simulink model "ANSFT_Euler"  (R2023a)
settings: Solver=ode1  StartTime=0.0  StopTime=60  FixedStep=0.01  RelTol=1e-3
undefined symbols (not defined in the file or in its folder): HDBK, Light, MIL, sigbuilder_block
libraries: simulink x4, matrix_library x3, aerolibutil x3, robotcorelib x2, aerolibanim x1, simulink_extras x1, sharedtransform x1, aerolibwind2 x1, sim3dlib x1, uavsim3dlib x1
(part 1 of 2)
settings Model: Creator=goliv  LastModifiedBy=Adan Daniel
settings OptimizationCC: ReuseModelBlockBuffer=off

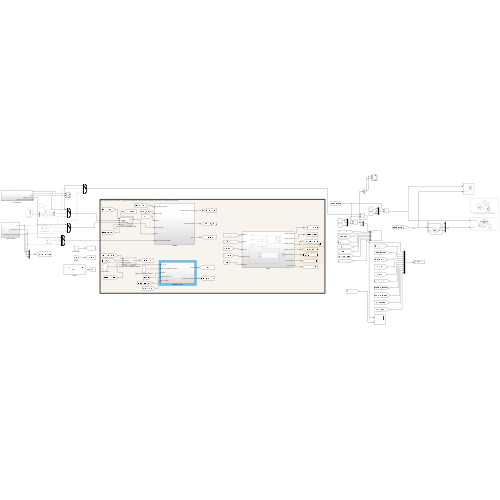
[thumbnail: Simulink's stored preview of the top-level diagram]
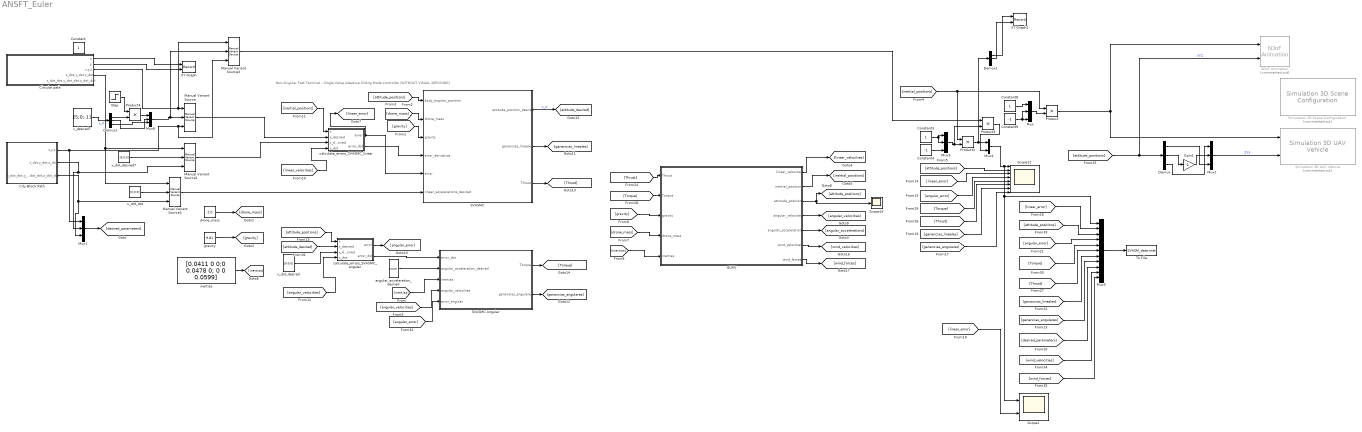
== system ANSFT_Euler ==
  note: Non-Singular Fast Terminal - Single Value Adaptive Sliding Mode Controller (WITHOUT VISUAL SERVOING)
  6DoF Animation : aerolibanim/6DoF Animation  Commented=on  u1=[0 4000 -2000 2000 -5000 -3000]  u2=0.1  u3=1.0  u4=[4000 0 -5000]  u5=Fixed position  u6=[2000 500 -3150]  u7=10  u8=on
  "Circular path " : Subsystem
  City Block Path : Subsystem
  Constant3 : Constant
  Constant4 : Constant  Value=-1
  Constant8 : Constant
  Constant9 : Constant  Value=-1
  Demux : Demux  Outputs=3
  Demux1 : Demux  Outputs=3
  Demux2 : Demux  Outputs=3
  Gain1 : Gain  Gain=-1
  Manual Variant Source{,1..3} (4 alike) : simulink/Signal Routing/Manual Variant Source  NumChoices=3  LabelModeActiveChoice=V_1
  Mux{,1..3,6} (5 alike) : Mux  Inputs=3
  Mux4 : Mux  Inputs=2
  Mux5 : Mux  Inputs=11
  Product{,2..4} (4 alike) : Product
  QUAV : Subsystem
  SVASMC : Subsystem
  SVASMC Angular : Subsystem
  Scope1 : Scope  NumInputPorts=2
  Scope12 : Scope  NumInputPorts=8
  Scope15 : Scope
  Simulation 3D Scene Configuration : sim3dlib/Simulation 3D Scene Configuration  Priority=0  Commented=on  ProjectFormat=Default Scenes  SceneDesc=US city block  ProjectName=C:\Program Files\MATLAB\R2023a\toolbox\shared\sim3d_projects\automotive_project\UE4\WindowsNoEditor\VehicleSimulation.exe  ScenePath=/Game/Maps/USCityBlock  EnableOpenDRIVE=off  vehTagList={'Scene Origin';'SimulinkVehicle1'}  vehTag=SimulinkVehicle1  OpVisEn=off  Ts=0.01  EnableWindow=on  EnableRemoteAccess=off  EnableWeather=off  SunAltitude=40.0  SunAzimuth=90  clouds=10  wind=1  fog=0  rain=0  EnableGeospatial=off  OriginHeight=200  OriginLatitude=40.744652  OriginLongitude=-73.988864  MapStyle=Aerial  AdditionalAssetIDs=[]  UseAdvancedSunSky=off  SolarTime=11  TimeZone=-5  Day=21  Month=9  Year=2022  UseDaylightSavingTime=on  DSTStartDay=10  DSTStartMonth=3  DSTEndDay=3  DSTEndMonth=11  DSTSwitchHour=2  sensorTag=MainCamera1  sensorId=1  sensorName=MainCamera1  mountLoc=Origin  offsetFlag=off  tmountOffset=[0, 0, 0]  rmountOffset=[0, 0, 0]  HorizontalResolution=1280  VerticalResolution=720  HorizontalFOV=60  mountPoint=[0 0 0]  mountOrientation=[0 0 0]  aMode=4  ID=1  GeoTrigger=Inactive
      settings: LibrarySourceBlock=uavsim3dlib/Simulation 3D Scene Configuration
  Simulation 3D UAV Vehicle : uavsim3dlib/Simulation 3D UAV Vehicle  Priority=-1  Commented=on  Mesh=Quadrotor  MeshPath=/MathWorksUAVContent/UAVs/HexaRotorUAV/HexaRotor.HexaRotor  Color=Black  ActorName=SimulinkVehicle1  UseGlobalFrame=off  InitialTranslation=[0 0 0]  InitialRotation=[0 0 0]  InitialTranslationGlobal=[0 0 0]  InitialGeoOrigin=[0 0 0]  InitialRotationGlobal=[0 0 0]  SampleTime=-1  ActorType=SimulinkVehicle  ID=1  aMode=4  ActorTag=SimulinkVehicle1
  Step : Step  Time=2  SampleTime=0
  To File : ToFile  Filename=SVASM_data.mat  SaveFormat=Timeseries
  XY Graph : Record  FileSettingsInternal="{\"entries\":[{\"content\":{\"excelSettings\":{\"content\":{},\"type\":\"Streamout.ExcelSettings\"}},\"type\":\"Streamout.FileSettingStorage\",\"uuid\":\"\"}],\"packageUris\":[\"http:\\/\\/schema.mathworks.com\\/mf0\\/streamout_blocks\\/R2020a\"],\"version\":\"1.0\"}"  Layout=[1 1]  SignalsInternal="{\"entries\":[{\"content\":{\"signals\":[{\"content\":{\"blockPath\":[],\"dimensions\":[1],\"domain\":\"\",\"lineColor\":\"#0072bd\",\"port\":1,\"sid\":[\"\"],\"signalID\":103,\"signalName\":\"Circular path :1\"},\"type\":\"RecordBlkView.Signal\",\"uuid\":\"\"},{\"content\":{\"blockPath\":[],\"dimensions\":[1],\"domain\":\"\",\"lineColor\":\"#d95319\",\"port\":2,\"sid\":[\"\"],\"signalID\":107,\"signalName\":\"Circular path :2\"},\"type\":\"RecordBlkView.Signal\",\"uuid\":\"\"}]},\"type\":\"RecordBlkView.InputSignals\",\"uuid\":\"\"}],\"packageUris\":[\"http:\\/\\/schema.mathworks.com\\/mf0\\/streamout_blocks\\/R2020a\"],\"version\":\"1.0\"}"  VisualizationBindings="{\"xyplotplugin\":{\"info\":[{\"series\":[],\"subplotID\":1}]}}"  CompatibilityTag=XY
  XY Graph1 : Record  FileSettingsInternal="{\"entries\":[{\"content\":{\"excelSettings\":{\"content\":{},\"type\":\"Streamout.ExcelSettings\"}},\"type\":\"Streamout.FileSettingStorage\",\"uuid\":\"\"}],\"packageUris\":[\"http:\\/\\/schema.mathworks.com\\/mf0\\/streamout_blocks\\/R2020a\"],\"version\":\"1.0\"}"  Layout=[1 1]  SignalsInternal="{\"entries\":[{\"content\":{\"signals\":[{\"content\":{\"blockPath\":[],\"dimensions\":[1,1],\"domain\":\"\",\"lineColor\":\"#edb120\",\"port\":1,\"sid\":[\"\"],\"signalID\":111,\"signalName\":\"Demux1:1\"},\"type\":\"RecordBlkView.Signal\",\"uuid\":\"\"},{\"content\":{\"blockPath\":[],\"dimensions\":[1,1],\"domain\":\"\",\"lineColor\":\"#7e2f8e\",\"port\":2,\"sid\":[\"\"],\"signalID\":115,\"signalName\":\"Demux1:2\"},\"type\":\"RecordBlkView.Signal\",\"uuid\":\"\"}]},\"type\":\"RecordBlkView.InputSignals\",\"uuid\":\"\"}],\"packageUris\":[\"http:\\/\\/schema.mathworks.com\\/mf0\\/streamout_blocks\\/R2020a\"],\"version\":\"1.0\"}"  VisualizationBindings="{\"xyplotplugin\":{\"info\":[{\"series\":[],\"subplotID\":1}]}}"  CompatibilityTag=XY
  angular_acceleration_desired : Constant  Value=[0;0;0]  VectorParams1D=off
  calculate_errors_SVASMC_angular : Subsystem
  calculate_errors_SVASMC_linear : Subsystem
  drone_mass : Constant  Value=2.0
  gravity : Constant  Value=9.81
  inertias : Constant  Value=[0.0411 0 0;0 0.0478 0; 0 0 0.0599]  VectorParams1D=off
  x_desired7 : Constant  Value=[5;0;-1]  VectorParams1D=off
  x_dot_desired : Constant  Value=[0;0;0]  VectorParams1D=off
  x_dot_desired7 : Constant  Value=[0;0;0]  VectorParams1D=off
  x_dot_dot : Constant  Value=[0;0;0]  VectorParams1D=off
  Constant : Constant  IOType=siggen
  wires:
  [ganancias_lineales] -> Scope12/7
  [inertias] -> SVASMC Angular/3(inertias)
  [inertial_positions] -> calculate_errors_SVASMC_linear/1(x)
  [Torque] -> Scope12/5
  SVASMC Angular/1(Torque) -> [Torque]
  [angular_error] -> SVASMC Angular/5(error_angular)
  [attitude_desired] -> calculate_errors_SVASMC_angular/2(x_desired)
  [Thrust] -> QUAV/1(Thrust)
  SVASMC Angular/2(ganancias_angulares) -> [ganancias_angulares]
  [drone_mass] -> QUAV/4(drone_mass)
  [attitude_positions] -> 6DoF Animation/2, Demux/1  "XYZ"
  [linear_error] -> Scope12/3
  SVASMC/2(ganancias_lineales) -> [ganancias_lineales]
  [attitude_positions] -> calculate_errors_SVASMC_angular/1(x)
  Constant9/1 -> Mux/2, Mux/3
  inertias/1 -> [inertias]
  [drone_mass] -> SVASMC/2(drone_mass)
  x_dot_desired/1 -> calculate_errors_SVASMC_angular/3(x_dot_desired)
  QUAV/5(angular_accelerations) -> [angular_accelerations]
  calculate_errors_SVASMC_linear/1(error) -> [linear_error], SVASMC/5(error)
  QUAV/1(linear_velocities) -> [linear_velocities]
  SVASMC/3(Thrust) -> [Thrust]
  [attitude_positions] -> SVASMC/1(body_angular_position)
  [angular_velocities] -> SVASMC Angular/4(angular_velocities)
  [linear_velocities] -> calculate_errors_SVASMC_linear/4(x_dot)
  [inertial_positions] -> Product2/1, Product/1
  QUAV/2(inertial_positions) -> [inertial_positions]
  drone_mass/1 -> [drone_mass]
  [attitude_positions] -> Scope12/2
  QUAV/4(angular_velocities) -> [angular_velocities]
  calculate_errors_SVASMC_angular/1(error) -> [angular_error]
  [Torque] -> QUAV/2(Torque)
  [inertias] -> QUAV/5(inertias)
  gravity/1 -> [gravity]
  Demux/3 -> Mux2/1
  Constant8/1 -> Mux/1
  [gravity] -> SVASMC/3(gravity)
  QUAV/3(attitude_positions) -> Scope15/1, [attitude_positions]
  calculate_errors_SVASMC_angular/2(error_dot) -> SVASMC Angular/1(error_dot)
  [ganancias_angulares] -> Scope12/8
  calculate_errors_SVASMC_linear/2(error_dot) -> SVASMC/4(error_derivative)
  [gravity] -> QUAV/3(gravity)
  Mux/1 -> Product/2
  Demux/2 -> Gain1/1
  SVASMC/1(attitude_position_desired) -> [attitude_desired]  "x_d"
  [angular_error] -> Scope12/4
  angular_acceleration_desired/1 -> SVASMC Angular/2(angular_acceleration_desired)
  [angular_velocities] -> calculate_errors_SVASMC_angular/4(x_dot)
  [linear_error] -> Scope1/2
  [Thrust] -> Scope12/6
  Product/1 -> 6DoF Animation/1, Simulation 3D UAV Vehicle/1
  Mux3/1 -> Product2/2, Product3/2
  Constant4/1 -> Mux3/3
  Constant3/1 -> Mux3/2, Mux3/1
  Manual Variant Source/1 -> calculate_errors_SVASMC_linear/2(x_desired)
  "Circular path "/1(x) -> XY Graph/1
  "Circular path "/2(y) -> XY Graph/2
  "Circular path "/3(x,y,z) -> Manual Variant Source3/1, Manual Variant Source/1
  "Circular path "/4(x_dot,y_dot,z_dot) -> Manual Variant Source2/1, Manual Variant Source1/1
  x_dot_desired7/1 -> Manual Variant Source1/2
  Manual Variant Source1/1 -> calculate_errors_SVASMC_linear/3(x_dot_desired)
  Product2/1 -> Mux4/1, Demux1/1
  Mux4/1 -> Scope1/1, Mux5/1, Scope12/1
  Product3/1 -> Mux4/2
  Demux1/1 -> XY Graph1/1
  Demux1/2 -> XY Graph1/2
  Mux5/1 -> To File/1
  City Block Path/1(x,y,z) -> Manual Variant Source3/3, Manual Variant Source/3, Mux1/1
  City Block Path/2(x_dot,y_dot,z_dot) -> Mux1/2, Manual Variant Source1/3
  City Block Path/3(x_dot_dot,y_dot_dot,z_dot_dot) -> Mux1/3, Manual Variant Source2/3
  Manual Variant Source3/1 -> Product3/1
  x_dot_dot/1 -> Manual Variant Source2/2
  Manual Variant Source2/1 -> SVASMC/6(linear_accelerations_desired)
  Step/1 -> Product4/1
  x_desired7/1 -> Demux2/1  "x_d"
  Demux2/1 -> Product4/2
  Product4/1 -> Mux6/1
  Demux2/2 -> Mux6/2
  Demux2/3 -> Mux6/3
  Mux6/1 -> Manual Variant Source/2, Manual Variant Source3/2
  Mux2/1 -> Simulation 3D UAV Vehicle/2  "ZYX"
  Demux/1 -> Mux2/3
  Gain1/1 -> Mux2/2
  [linear_error] -> Mux5/2
  [attitude_positions] -> Mux5/3
  [angular_error] -> Mux5/4
  [Torque] -> Mux5/5
  [Thrust] -> Mux5/6
  [ganancias_lineales] -> Mux5/7
  [ganancias_angulares] -> Mux5/8
  Mux1/1 -> [desired_parameters]
  [desired_parameters] -> Mux5/9
  QUAV/6(wind_velocities) -> [wind_velocities]
  QUAV/7(wind_forces) -> [wind_forces]
  [wind_velocities] -> Mux5/10
  [wind_forces] -> Mux5/11

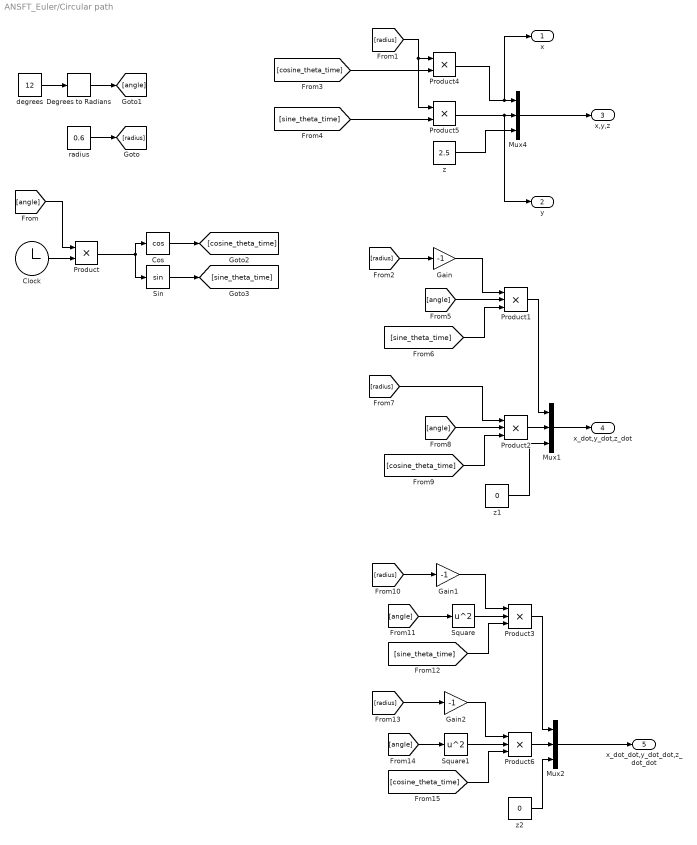
== system ANSFT_Euler/Circular path  ==
  Clock : Clock
  Cos : Trigonometry  Operator=cos
  Degrees to Radians : simulink_extras/Transformations/Degrees to Radians
  Gain : Gain  Gain=-1
  Gain1 : Gain  Gain=-1
  Gain2 : Gain  Gain=-1
  Mux1 : Mux  Inputs=3
  Mux2 : Mux  Inputs=3
  Mux4 : Mux  Inputs=3
  Product : Product
  Product{1..3,6} (4 alike) : Product  Inputs=3
  Product4 : Product
  Product5 : Product
  Sin : Trigonometry
  Square : Math  Operator=square
  Square1 : Math  Operator=square
  degrees : Constant  Value=12
  radius : Constant  Value=0.6
  z : Constant  Value=2.5
  z1 : Constant  Value=0
  z2 : Constant  Value=0
  x : Outport
  y : Outport  Port=2
  x,y,z : Outport  Port=3
  x_dot,y_dot,z_dot : Outport  Port=4
  x_dot_dot,y_dot_dot,z_dot_dot : Outport  Port=5
  wires:
  Mux4/1 -> x,y,z/1
  Product4/1 -> x/1, Mux4/1
  Product5/1 -> y/1, Mux4/2
  degrees/1 -> Degrees to Radians/1
  Clock/1 -> Product/2
  radius/1 -> [radius]
  Degrees to Radians/1 -> [angle]
  [radius] -> Product5/1, Product4/1
  [angle] -> Product/1
  [radius] -> Gain/1
  Product/1 -> Cos/1, Sin/1
  Cos/1 -> [cosine_theta_time]
  Sin/1 -> [sine_theta_time]
  [cosine_theta_time] -> Product4/2
  [sine_theta_time] -> Product5/2
  Gain/1 -> Product1/1
  [angle] -> Product1/2
  [sine_theta_time] -> Product1/3
  [cosine_theta_time] -> Product2/3
  [angle] -> Product2/2
  [radius] -> Product2/1
  Product1/1 -> Mux1/1
  Product2/1 -> Mux1/2
  Mux1/1 -> x_dot,y_dot,z_dot/1
  Mux2/1 -> x_dot_dot,y_dot_dot,z_dot_dot/1
  Product6/1 -> Mux2/2
  Product3/1 -> Mux2/1
  [radius] -> Gain2/1
  [angle] -> Square1/1
  [cosine_theta_time] -> Product6/3
  [sine_theta_time] -> Product3/3
  [angle] -> Square/1
  Gain1/1 -> Product3/1
  [radius] -> Gain1/1
  z/1 -> Mux4/3
  Gain2/1 -> Product6/1
  Square/1 -> Product3/2
  Square1/1 -> Product6/2
  z1/1 -> Mux1/3
  z2/1 -> Mux2/3

== system ANSFT_Euler/City Block Path ==
  Clock : Clock
  Polynomial Trajectory : robotcorelib/Polynomial Trajectory  WaypointSource=Internal  Waypoints=[0, 0, 0; 0 0 -15; 70 0 -15; 70 110 -15; 170 110 -15; 170 110 0]'  TimePoints=[0, 10, 30, 60, 90, 110]  TimeInterval=[ 1, 4 ]  Method=Cubic Polynomial  ParameterSource=Internal  VelocityBoundaryCondition=zeros( 3, 6 )  AccelerationBoundaryCondition=zeros( 2, 5 )  SimulateUsing=Interpreted execution
  Scope2 : Scope  NumInputPorts=3
  Trapezoidal Velocity Profile Trajectory : robotcorelib/Trapezoidal Velocity Profile Trajectory  Commented=on  WaypointSource=Internal  Waypoints=[0, 0, 0; 30 0 -10; 70 0 -10; 70 110 -10; 170 110 -10]'  NumParams=1  Parameter1=Peak Velocity  Parameter2=End Time  ParameterSource=Internal  PeakVelocity=[2.5; 2.5; 4]  Acceleration=[ 1; 2 ]  EndTime=[1, 30, 30, 50, 50]  AccelTime=[ 1; 2 ]  SimulateUsing=Interpreted execution
  x,y,z : Outport
  x_dot,y_dot,z_dot : Outport  Port=2
  x_dot_dot,y_dot_dot,z_dot_dot : Outport  Port=3
  wires:
  Clock/1 -> Polynomial Trajectory/1
  Polynomial Trajectory/2 -> Scope2/2, x_dot,y_dot,z_dot/1
  Polynomial Trajectory/1 -> Scope2/1, x,y,z/1
  Polynomial Trajectory/3 -> Scope2/3, x_dot_dot,y_dot_dot,z_dot_dot/1

== system ANSFT_Euler/QUAV ==
  Thrust : Inport
  Torque : Inport  Port=2
  gravity : Inport  Port=3
  drone_mass : Inport  Port=4
  inertias : Inport  Port=5
  Subsystem : Subsystem
  linear dynamics : Subsystem
  linear_velocities : Outport
  inertial_positions : Outport  Port=2
  attitude_positions : Outport  Port=3
  angular_velocities : Outport  Port=4
  angular_accelerations : Outport  Port=5
  wind_velocities : Outport  Port=6
  wind_forces : Outport  Port=7
  wires:
  Thrust/1 -> linear dynamics/1(Thrust)
  drone_mass/1 -> linear dynamics/4(drone_mass)
  linear dynamics/2(linear_velocities) -> linear_velocities/1
  Torque/1 -> Subsystem/1(Torque)
  gravity/1 -> linear dynamics/3(gravity)
  linear dynamics/3(inertial_positions) -> inertial_positions/1
  inertias/1 -> Subsystem/2(inertias)
  Subsystem/2(angular_velocities) -> linear dynamics/5(angular_velocities), angular_velocities/1
  Subsystem/1(attitude_positions) -> linear dynamics/2(attitude_positions), attitude_positions/1
  Subsystem/3(angular_accelerations) -> angular_accelerations/1
  linear dynamics/4(wind_velocities) -> wind_velocities/1
  linear dynamics/5(wind_forces) -> wind_forces/1

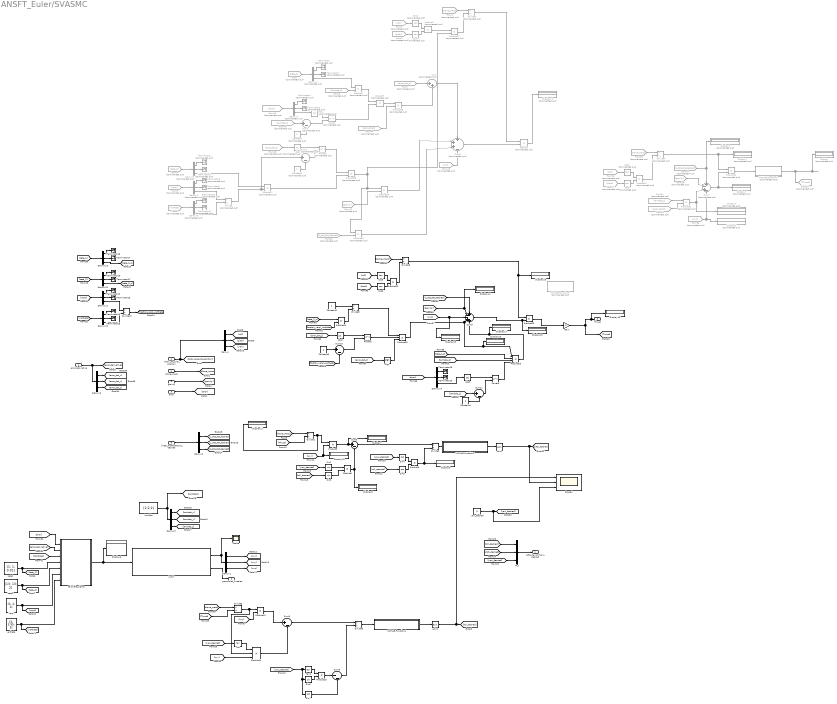
== system ANSFT_Euler/SVASMC ==
  body_angular_position : Inport
  drone_mass : Inport  Port=2
  gravity : Inport  Port=3
  error_derivative : Inport  Port=4
  error : Inport  Port=5
  linear_accelerations_desired : Inport  Port=6
  Abs : Abs  Commented=on  SaturateOnIntegerOverflow=off
  Abs1 : Abs  Commented=on  SaturateOnIntegerOverflow=off
  Abs2 : Abs  SaturateOnIntegerOverflow=off
  Abs3 : Abs  SaturateOnIntegerOverflow=off
  Asin1 : Trigonometry  Operator=asin
  Asin2 : Trigonometry  Operator=asin
  Constant : Constant  Commented=on
  Constant1 : Constant  Commented=on
  Constant2 : Constant
  Constant3 : Constant  Value=2
  Constant4 : Constant
  Cos{1..4} (4 alike) : Trigonometry  Commented=on  Operator=cos
  Cos5 : Trigonometry  Operator=cos
  Cos6 : Trigonometry  Operator=cos
  Demux{,1..3,6,10..14} (10 alike) : Demux  Outputs=3
  Demux{4..5,7..9} (5 alike) : Demux  Commented=on  Outputs=3
  Display{,1..5,12} (7 alike) : Display  Commented=on
  Display{6..11,13..19} (13 alike) : Display
  Divide : Product  Commented=on  Inputs=*/
  Divide{1,3,5..6,8..10} (7 alike) : Product  Inputs=*/
  Divide4 : Product  Commented=on  Inputs=*/
  Divide7 : Product  Commented=on  Inputs=*/
  From : From  Commented=on  GotoTag=zeta_1
  From1 : From  Commented=on  GotoTag=drone_mass
  From2 : From  Commented=on  GotoTag=roll
  From25 : From  Commented=on  GotoTag=drone_mass
  From26 : From  Commented=on  GotoTag=roll
  From27 : From  Commented=on  GotoTag=pitch
  From{7,28,44..45} (4 alike) : From  Commented=on  GotoTag=error_dot_z
  From29 : From  Commented=on  GotoTag=gravity
  From3 : From  Commented=on  GotoTag=pitch
  From30 : From  Commented=on  GotoTag=z_dot_dot_desired
  From31 : From  Commented=on  GotoTag=lambda_z
  From36 : From  Commented=on  GotoTag=uvz
  From4 : From  Commented=on  GotoTag=zeta_2
  From42 : From  Commented=on  GotoTag=error
  From43 : From  Commented=on  GotoTag=lambda_z
  From46 : From  Commented=on  GotoTag=gravity
  From47 : From  Commented=on  GotoTag=z_dot_dot_desired
  From48 : From  Commented=on  GotoTag=uvz
  From5 : From  Commented=on  GotoTag=varpi
  From6 : From  Commented=on  GotoTag=vartheta
  From8 : From  Commented=on  GotoTag=lambda_z
  Gain : Gain  Gain=-1
  Goto33 : Goto  Commented=on  GotoTag=Thrust
  MATLAB Function2 : MATLAB Function  TreatAsAtomicUnit=on
  MATLAB Function3 : MATLAB Function  Commented=on  TreatAsAtomicUnit=on
  MATLAB Function4 : MATLAB Function  TreatAsAtomicUnit=on
  MATLAB Function5 : MATLAB Function  Commented=on  TreatAsAtomicUnit=on
  Mux : Mux  Inputs=3
  Power : Math  Commented=on  Operator=pow
  Power1 : Math  Commented=on  Operator=pow
  Power2 : Math  Operator=pow
  Power3 : Math  Operator=pow
  Product{,1..2,7,10..12,16..21} (13 alike) : Product  Commented=on
  Product{3,8..9,13,15,22..24} (8 alike) : Product
  Product14 : Product  Inputs=3
  Product25 : Product  Inputs=3
  Product26 : Product  Inputs=4
  Scope : Scope
  Scope1 : Scope  NumInputPorts=3
  Sign : Signum
  Sin2 : Trigonometry
  Sin3 : Trigonometry
  Sin4 : Trigonometry  Operator=cos
  Sin5 : Trigonometry  Operator=cos
  Sin6 : Trigonometry
  Sin7 : Trigonometry  Operator=cos
  Sum : Sum  Commented=on  Inputs=|++
  Sum1 : Sum  Commented=on  Inputs=|+-
  Sum{3,5,10..11} (4 alike) : Sum  Inputs=|+-
  Sum2 : Sum  Commented=on  Inputs=|+-
  Sum6 : Sum  Commented=on  Inputs=+++-
  Sum7 : Sum  Commented=on  Inputs=+-+-
  Sum8 : Sum  Inputs=|--
  Sum9 : Sum  Inputs=+--++
  Tan : Trigonometry  Operator=tan
  Tan1 : Trigonometry  Operator=tan
  Terminator{,1..9} (10 alike) : Terminator  Commented=on
  Terminator{10..19} (10 alike) : Terminator
  calculate_sigma : Subsystem
  lambda : Constant  Value=[2;2;2]  VectorParams1D=off
  u_aux : Subsystem
  varpi : Constant  Value=[4; 4; 4]  VectorParams1D=off
  vartheta : Constant  Value=[3; 3.95; 3]  VectorParams1D=off
  yaw_desired : Constant  Value=0
  zeta1 : Constant  Value=[1; 1; 0.01]  VectorParams1D=off
  zeta2 : Constant  Value=[13; 13; 2]  VectorParams1D=off
  attitude_position_desired : Outport
  ganancias_lineales : Outport  Port=2
  Thrust : Outport  Port=3
  wires:
  body_angular_position/1 -> Demux/1, [body_angular_position]
  drone_mass/1 -> [drone_mass]
  gravity/1 -> [gravity]
  error_derivative/1 -> Demux6/1, [error_derivative]
  error/1 -> [error]
  linear_accelerations_desired/1 -> Demux2/1
  Demux/1 -> [roll]
  Demux/2 -> [pitch]
  Demux/3 -> [yaw]
  u_aux/1(u_aux) -> Demux1/1, Scope/1
  Demux1/3 -> [uvz]
  Demux1/2 -> [uvy]
  Demux1/1 -> [uvx]
  Demux2/3 -> [z_dot_dot_desired]
  Demux2/2 -> [y_dot_dot_desired]
  Demux2/1 -> [x_dot_dot_desired]
  Demux3/1 -> [lambda_x]
  Demux3/2 -> [lambda_y]
  Demux3/3 -> [lambda_z]
  [drone_mass] -> Divide1/1
  Divide1/1 -> Display11/1, Product3/1
  [uvx] -> Product3/2, Display10/1
  Product3/1 -> Display7/1, Sum3/1
  [yaw_desired] -> Sin2/1
  Sin2/1 -> Product8/1
  [roll_desired] -> Sin3/1
  Sin3/1 -> Product8/2
  Product8/1 -> Display8/1, Sum3/2
  Sum3/1 -> Divide3/1
  [yaw_desired] -> Sin4/1
  [roll_desired] -> Sin5/1
  Sin4/1 -> Product9/1
  Sin5/1 -> Product9/2
  Product9/1 -> Display9/1, Divide3/2
  [roll_desired] -> Mux/1
  [pitch_desired] -> Mux/2
  [yaw_desired] -> Mux/3
  Mux/1 -> attitude_position_desired/1
  MATLAB Function2/1(final_pitch_parameter) -> Asin1/1
  Divide3/1 -> MATLAB Function2/1(pitch_parameter)
  From26/1 -> Cos2/1
  MATLAB Function3/1(final_thrust) -> Display/1, Goto33/1
  From31/1 -> Product12/1
  Product10/1 -> Divide4/2
  Cos2/1 -> Product10/1
  From25/1 -> Divide4/1
  Cos3/1 -> Product10/2
  From27/1 -> Cos3/1
  From47/1 -> Sum7/1, Display3/1
  From29/1 -> Sum7/2
  Product12/1 -> Display4/1, Sum7/3
  From36/1 -> Display5/1, Sum7/4
  Sum7/1 -> Display2/1, Product11/2
  Divide4/1 -> Product11/1, Display1/1
  Product11/1 -> MATLAB Function3/1(thrust)
  Demux6/1 -> [error_dot_x]
  Demux6/2 -> [error_dot_y]
  Demux6/3 -> [error_dot_z]
  From28/1 -> Product12/2
  yaw_desired/1 -> Scope1/3, [yaw_desired]  "yaw desired"
  MATLAB Function4/1(final_roll_parameter) -> Asin2/1
  [drone_mass] -> Divide5/1
  Divide5/1 -> Product14/2, Product13/1
  [uvy] -> Product13/2
  Product13/1 -> Sum5/1
  [yaw_desired] -> Tan/1
  Tan/1 -> Product14/1
  [uvx] -> Product14/3
  Product14/1 -> Sum5/2
  Sum5/1 -> Divide6/1
  [yaw_desired] -> Sin7/1, Sin6/1, Tan1/1
  Tan1/1 -> Product15/1
  Sin6/1 -> Product15/2
  Product15/1 -> Sum8/1
  Sin7/1 -> Sum8/2
  Sum8/1 -> Divide6/2
  Divide6/1 -> MATLAB Function4/1(roll_parameter)
  Asin1/1 -> Scope1/2, [pitch_desired]  "pitch desired"
  Asin2/1 -> Scope1/1, [roll_desired]  "roll desired"
  u_aux/2(k_lineales) -> ganancias_lineales/1
  [error] -> calculate_sigma/1(error1)
  [error_derivative] -> calculate_sigma/2(error_derivative)
  lambda/1 -> [lambdas], Demux3/1
  calculate_sigma/1(sigma_lineales) -> Display6/1, u_aux/1(sigma_lineal)
  varpi/1 -> [varpi], calculate_sigma/6(varpi)
  zeta1/1 -> [zeta_1], calculate_sigma/4(zeta1)
  vartheta/1 -> [vartheta], calculate_sigma/7(vartheta)
  zeta2/1 -> [zeta_2], calculate_sigma/5(zeta2)
  [lambdas] -> calculate_sigma/3(lambda)
  From3/1 -> Cos4/1
  Cos4/1 -> Product1/2
  From1/1 -> Divide7/1
  Cos1/1 -> Product1/1
  From2/1 -> Cos1/1
  Divide7/1 -> Product/1
  From/1 -> Demux4/1
  Demux4/1 -> Terminator/1
  Demux4/2 -> Terminator1/1
  Demux5/2 -> Terminator3/1
  Demux5/1 -> Terminator2/1
  From4/1 -> Demux5/1
  Demux4/3 -> Product2/1
  From8/1 -> Product2/2
  From7/1 -> Sum/1
  Demux7/2 -> Terminator5/1
  Demux7/1 -> Terminator4/1
  From42/1 -> Demux7/1
  Demux7/3 -> Abs/1
  Abs/1 -> Power/1
  From43/1 -> Sum1/1
  Constant/1 -> Sum1/2
  Sum1/1 -> Power/2
  Product2/1 -> Product7/1
  Power/1 -> Product7/2
  Product7/1 -> Product16/1
  From44/1 -> Product16/2
  Product16/1 -> Sum/2
  From5/1 -> Demux8/1
  Demux8/1 -> Terminator6/1
  Demux8/2 -> Terminator7/1
  Demux9/2 -> Terminator9/1
  Demux9/1 -> Terminator8/1
  From6/1 -> Demux9/1
  Demux8/3 -> Divide/1
  Demux9/3 -> Divide/2
  Divide/1 -> Sum2/1, Product17/2
  Demux5/3 -> Product17/1
  From45/1 -> Abs1/1
  Abs1/1 -> Power1/1
  Sum2/1 -> Power1/2
  Constant1/1 -> Sum2/2
  Product17/1 -> Product18/2
  Power1/1 -> Product18/1
  Sum/1 -> Sum6/1  "iota"
  Product18/1 -> Product21/2, Product20/1, Product19/1  "t"
  From46/1 -> Product19/2
  Product19/1 -> Sum6/2
  From30/1 -> Product20/2
  Product20/1 -> Sum6/3
  From48/1 -> Sum6/4
  Sum6/1 -> Product/2
  Product/1 -> Display12/1
  Product1/1 -> Product21/1
  Product21/1 -> Divide7/2
  [vartheta] -> Demux12/1
  Demux12/1 -> Terminator14/1
  Demux12/2 -> Terminator15/1
  Demux11/2 -> Terminator13/1
  Demux11/1 -> Terminator12/1
  [varpi] -> Demux11/1
  [zeta_2] -> Demux10/1
  Demux10/1 -> Terminator10/1
  Demux10/2 -> Terminator11/1
  [roll] -> Cos5/1
  Cos5/1 -> Product22/1
  Cos6/1 -> Product22/2
  [pitch] -> Cos6/1
  [drone_mass] -> Divide8/1
  Product22/1 -> Divide8/2
  Divide8/1 -> Display18/1, Product23/1
  [z_dot_dot_desired] -> Sum9/1
  [gravity] -> Display14/1, Sum9/2
  [uvz] -> Display15/1, Sum9/3
  Demux13/2 -> Terminator17/1
  Demux13/1 -> Terminator16/1
  [zeta_1] -> Demux13/1
  Demux10/3 -> [zeta_2_z]
  Demux13/3 -> [zeta_1_z]
  Demux11/3 -> Divide10/1
  Demux12/3 -> Divide10/2
  Constant2/1 -> Divide9/1
  Divide10/1 -> [fraction_varpi_vartheta]
  [zeta_2_z] -> Product24/1
  [fraction_varpi_vartheta] -> Product24/2
  Product24/1 -> Divide9/2
  [error_dot_z] -> Abs2/1
  Divide9/1 -> Product25/1
  Abs2/1 -> Power2/1
  Constant3/1 -> Sum10/1
  [fraction_varpi_vartheta] -> Sum10/2
  Sum10/1 -> Power2/2
  Power2/1 -> Product25/2
  [error_dot_z] -> Sign/1
  Sign/1 -> Product25/3
  Product25/1 -> Display16/1, Product26/1, Sum9/4
  [zeta_1_z] -> Product26/2
  [lambda_z] -> Product26/3
  Power3/1 -> Product26/4
  Abs3/1 -> Power3/1
  [error] -> Demux14/1
  Demux14/1 -> Terminator18/1
  Demux14/2 -> Terminator19/1
  Demux14/3 -> Abs3/1
  [lambda_z] -> Sum11/1
  Constant4/1 -> Sum11/2
  Sum11/1 -> Power3/2
  Product26/1 -> Display17/1, Sum9/5
  Sum9/1 -> Display19/1, Product23/2
  [Thrust] -> Divide5/2
  [Thrust] -> Divide1/2
  Product23/1 -> Gain/1
  Gain/1 -> [Thrust], Display13/1, Thrust/1

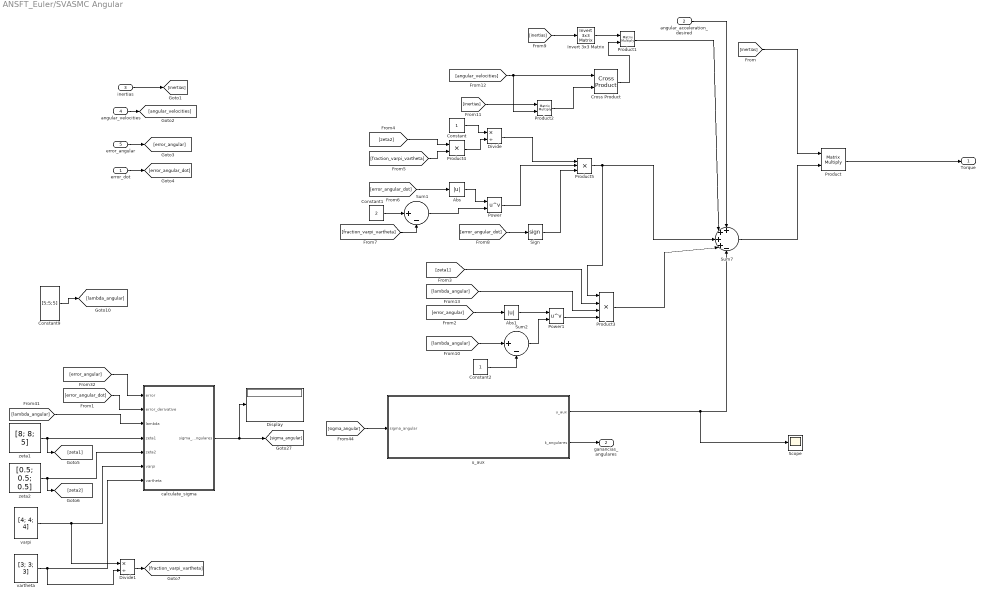
== system ANSFT_Euler/SVASMC Angular ==
  error_dot : Inport
  angular_acceleration_desired : Inport  Port=2
  inertias : Inport  Port=3
  angular_velocities : Inport  Port=4
  error_angular : Inport  Port=5
  Abs : Abs  SaturateOnIntegerOverflow=off
  Abs1 : Abs  SaturateOnIntegerOverflow=off
  Constant : Constant
  Constant1 : Constant  Value=2
  Constant2 : Constant
  Constant9 : Constant  Value=[5;5;5]  VectorParams1D=off
  Cross Product : matrix_library/Cross Product
  Display : Display
  Divide : Product  Inputs=*/
  Divide1 : Product  Inputs=*/
  Invert 3x3 Matrix : aerolibutil/Invert  3x3 Matrix
  Power : Math  Operator=pow
  Power1 : Math  Operator=pow
  Product : Product  Multiplication=Matrix(*)
  Product1 : Product  Multiplication=Matrix(*)
  Product2 : Product  Multiplication=Matrix(*)
  Product3 : Product  Inputs=4
  Product4 : Product
  Product5 : Product  Inputs=3
  Scope : Scope
  Sign : Signum
  Sum1 : Sum  Inputs=|+-
  Sum2 : Sum  Inputs=|+-
  Sum7 : Sum  Inputs=++++-
  calculate_sigma : Subsystem
  u_aux : Subsystem
  varpi : Constant  Value=[4; 4; 4]  VectorParams1D=off
  vartheta : Constant  Value=[3; 3; 3]  VectorParams1D=off
  zeta1 : Constant  Value=[8; 8; 5]  VectorParams1D=off
  zeta2 : Constant  Value=[0.5; 0.5; 0.5]  VectorParams1D=off
  Torque : Outport
  ganancias_angulares : Outport  Port=2
  wires:
  [angular_velocities] -> Product2/2, Cross Product/1
  [inertias] -> Product2/1
  [inertias] -> Product/1
  u_aux/1(u_aux) -> Sum7/5, Scope/1
  [inertias] -> Invert 3x3 Matrix/1
  Sum7/1 -> Product/2
  Product2/1 -> Cross Product/2
  Constant9/1 -> [lambda_angular]
  [sigma_angular] -> u_aux/1(sigma_angular)
  Cross Product/1 -> Product1/2
  Invert 3x3 Matrix/1 -> Product1/1
  inertias/1 -> [inertias]
  angular_velocities/1 -> [angular_velocities]
  calculate_sigma/1(sigma_angulares) -> Display/1, [sigma_angular]
  error_angular/1 -> [error_angular]
  error_dot/1 -> [error_angular_dot]
  u_aux/2(k_angulares) -> ganancias_angulares/1
  [error_angular] -> calculate_sigma/1(error)
  [error_angular_dot] -> calculate_sigma/2(error_derivative)
  [lambda_angular] -> calculate_sigma/3(lambda)
  vartheta/1 -> Divide1/2, calculate_sigma/7(vartheta)
  varpi/1 -> Divide1/1, calculate_sigma/6(varpi)
  zeta2/1 -> [zeta2], calculate_sigma/5(zeta2)
  zeta1/1 -> [zeta1], calculate_sigma/4(zeta1)
  angular_acceleration_desired/1 -> Sum7/1
  Product1/1 -> Sum7/2
  Constant/1 -> Divide/1
  Divide1/1 -> [fraction_varpi_vartheta]
  [fraction_varpi_vartheta] -> Product4/2
  [zeta2] -> Product4/1
  Product4/1 -> Divide/2
  Divide/1 -> Product5/1
  [error_angular_dot] -> Abs/1
  Abs/1 -> Power/1
  Constant1/1 -> Sum1/1
  [fraction_varpi_vartheta] -> Sum1/2
  Sum1/1 -> Power/2
  Power/1 -> Product5/2
  [error_angular_dot] -> Sign/1
  Sign/1 -> Product5/3
  Product5/1 -> Product3/1, Sum7/3
  [error_angular] -> Abs1/1
  Abs1/1 -> Power1/1
  [lambda_angular] -> Sum2/1
  Constant2/1 -> Sum2/2
  Sum2/1 -> Power1/2
  [zeta1] -> Product3/2
  [lambda_angular] -> Product3/3
  Power1/1 -> Product3/4
  Product3/1 -> Sum7/4
  Product/1 -> Torque/1

== system ANSFT_Euler/calculate_errors_SVASMC_angular ==
  x : Inport
  x_desired : Inport  Port=2
  x_dot_desired : Inport  Port=3
  x_dot : Inport  Port=4
  Display : Display
  Display1 : Display
  Display2 : Display
  Sum : Sum  Inputs=|+-
  Sum1 : Sum  Inputs=|+-
  error : Outport
  error_dot : Outport  Port=2
  wires:
  Sum1/1 -> error_dot/1
  Sum/1 -> Display/1, error/1
  x/1 -> Display2/1, Sum/2
  x_desired/1 -> Display1/1, Sum/1
  x_dot/1 -> Sum1/2
  x_dot_desired/1 -> Sum1/1

== system ANSFT_Euler/calculate_errors_SVASMC_linear ==
  x : Inport
  x_desired : Inport  Port=2
  x_dot_desired : Inport  Port=3
  x_dot : Inport  Port=4
  Display : Display
  Display1 : Display
  Sum : Sum  Inputs=|+-
  Sum1 : Sum  Inputs=|+-
  error : Outport
  error_dot : Outport  Port=2
  wires:
  x_dot_desired/1 -> Sum1/1
  x_dot/1 -> Sum1/2
  x_desired/1 -> Display/1, Sum/1
  x/1 -> Sum/2, Display1/1
  Sum/1 -> error/1
  Sum1/1 -> error_dot/1

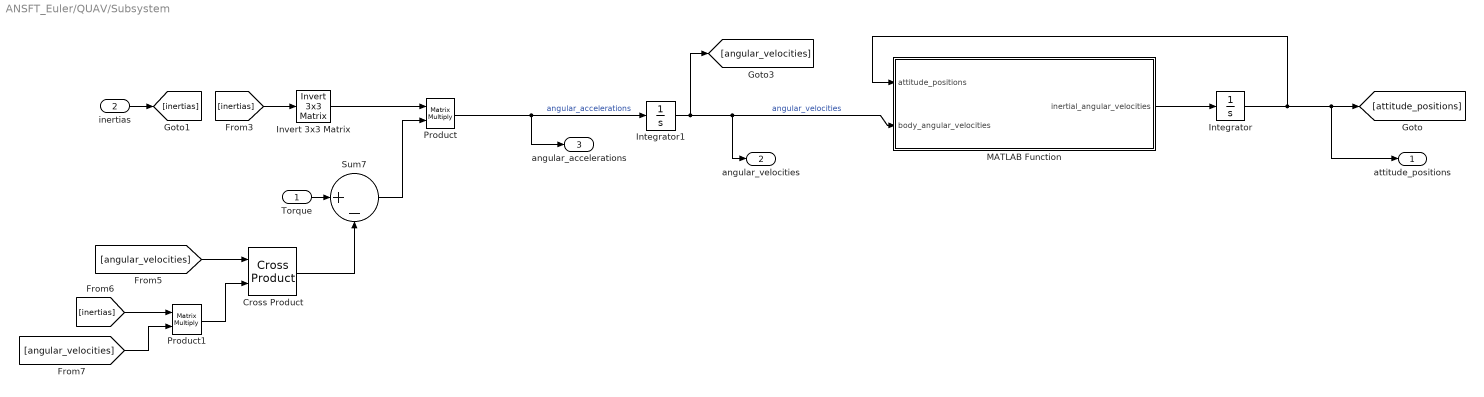
== system ANSFT_Euler/QUAV/Subsystem ==
  Torque : Inport
  inertias : Inport  Port=2
  Cross Product : matrix_library/Cross Product
  Integrator : Integrator  InitialCondition=[0;-0.0;-0.0]
  Integrator1 : Integrator  InitialCondition=[0;0;0]
  Invert 3x3 Matrix : aerolibutil/Invert  3x3 Matrix
  MATLAB Function : MATLAB Function  TreatAsAtomicUnit=on
  Product : Product  Multiplication=Matrix(*)
  Product1 : Product  Multiplication=Matrix(*)
  Sum7 : Sum  Inputs=|+-
  attitude_positions : Outport
  angular_velocities : Outport  Port=2
  angular_accelerations : Outport  Port=3
  wires:
  Torque/1 -> Sum7/1
  Sum7/1 -> Product/2
  Product/1 -> angular_accelerations/1, Integrator1/1  "angular_accelerations"
  [inertias] -> Invert 3x3 Matrix/1
  [angular_velocities] -> Cross Product/1
  Invert 3x3 Matrix/1 -> Product/1
  [angular_velocities] -> Product1/2
  Integrator/1 -> MATLAB Function/1(attitude_positions), attitude_positions/1, [attitude_positions]
  Product1/1 -> Cross Product/2
  Integrator1/1 -> [angular_velocities], angular_velocities/1, MATLAB Function/2(body_angular_velocities)  "angular_velocities"
  [inertias] -> Product1/1
  Cross Product/1 -> Sum7/2
  inertias/1 -> [inertias]
  MATLAB Function/1(inertial_angular_velocities) -> Integrator/1

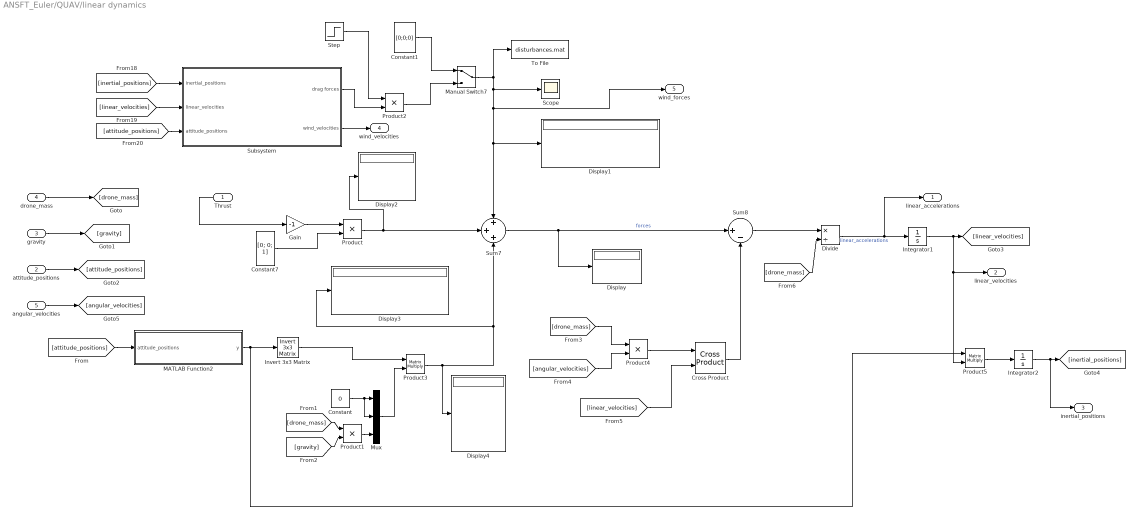
== system ANSFT_Euler/QUAV/linear dynamics ==
  Thrust : Inport
  attitude_positions : Inport  Port=2
  gravity : Inport  Port=3
  drone_mass : Inport  Port=4
  angular_velocities : Inport  Port=5
  Constant : Constant  Value=0
  Constant1 : Constant  Value=[0;0;0]  VectorParams1D=off
  Constant7 : Constant  Value=[0; 0; 1]  VectorParams1D=off
  Cross Product : matrix_library/Cross Product
  Display{,1..4} (5 alike) : Display
  Divide : Product  Inputs=*/
  Gain : Gain  Gain=-1
  Integrator1 : Integrator  InitialCondition=[0;0;0]
  Integrator2 : Integrator  InitialCondition=[0;0;0]
  Invert 3x3 Matrix : aerolibutil/Invert  3x3 Matrix
  MATLAB Function2 : MATLAB Function  TreatAsAtomicUnit=on
  Manual Switch7 : ManualSwitch
  Mux : Mux  Inputs=3
  Product{,1..2,4} (4 alike) : Product
  Product3 : Product  Multiplication=Matrix(*)
  Product5 : Product  Multiplication=Matrix(*)
  Scope : Scope
  Step : Step  Time=20  SampleTime=0
  Subsystem : Subsystem
  Sum7 : Sum  Inputs=+++
  Sum8 : Sum  Inputs=|+-
  To File : ToFile  Filename=disturbances.mat  SaveFormat=Timeseries
  linear_accelerations : Outport
  linear_velocities : Outport  Port=2
  inertial_positions : Outport  Port=3
  wind_velocities : Outport  Port=4
  wind_forces : Outport  Port=5
  wires:
  Sum7/1 -> Display/1, Sum8/1  "forces"
  Cross Product/1 -> Sum8/2
  [drone_mass] -> Divide/2
  [angular_velocities] -> Product4/2
  Sum8/1 -> Divide/1
  Integrator2/1 -> inertial_positions/1, [inertial_positions]
  Mux/1 -> Product3/2
  MATLAB Function2/1(y) -> Invert 3x3 Matrix/1, Product5/1
  Product4/1 -> Cross Product/1
  Constant7/1 -> Product/2
  Integrator1/1 -> linear_velocities/1, Product5/2, [linear_velocities]
  Product5/1 -> Integrator2/1
  [drone_mass] -> Product4/1
  Divide/1 -> linear_accelerations/1, Integrator1/1  "linear_accelerations"
  [linear_velocities] -> Cross Product/2
  attitude_positions/1 -> [attitude_positions]
  [attitude_positions] -> MATLAB Function2/1(attitude_positions)
  gravity/1 -> [gravity]
  drone_mass/1 -> [drone_mass]
  angular_velocities/1 -> [angular_velocities]
  [drone_mass] -> Product1/1
  [gravity] -> Product1/2
  Product1/1 -> Mux/3
  Constant/1 -> Mux/2, Mux/1
  Invert 3x3 Matrix/1 -> Product3/1
  Constant1/1 -> Manual Switch7/1
  Manual Switch7/1 -> To File/1, wind_forces/1, Display1/1, Sum7/1, Scope/1
  [inertial_positions] -> Subsystem/1(inertial_positions)
  [linear_velocities] -> Subsystem/2(linear_velocities)
  [attitude_positions] -> Subsystem/3(attitude_positions)
  Product3/1 -> Display4/1, Display3/1, Sum7/3
  Product/1 -> Display2/1, Sum7/2
  Thrust/1 -> Gain/1
  Subsystem/1("drag forces ") -> Product2/2
  Product2/1 -> Manual Switch7/2
  Step/1 -> Product2/1
  Gain/1 -> Product/1
  Subsystem/2(wind_velocities) -> wind_velocities/1

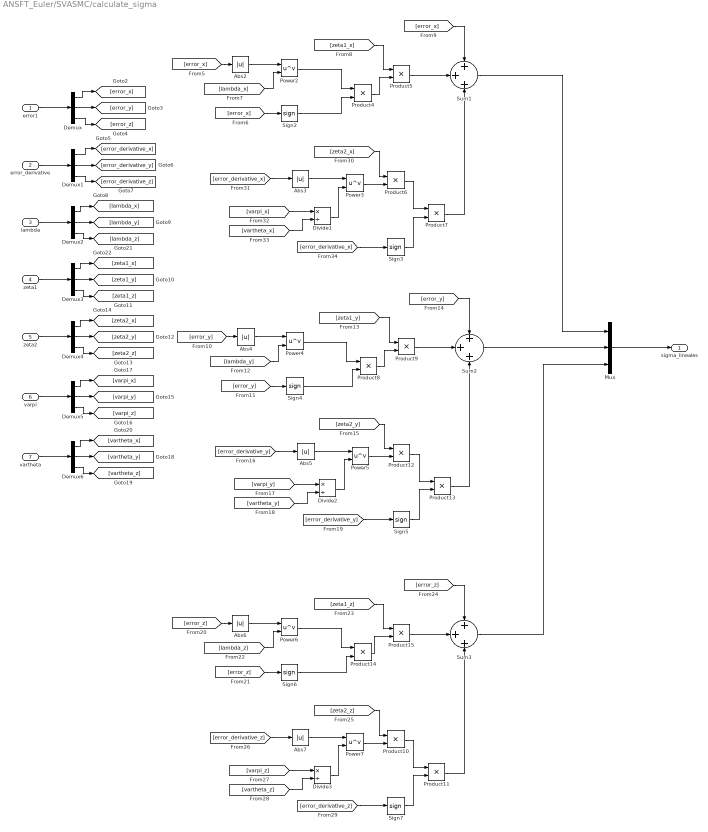
== system ANSFT_Euler/SVASMC/calculate_sigma ==
  error1 : Inport
  error_derivative : Inport  Port=2
  lambda : Inport  Port=3
  zeta1 : Inport  Port=4
  zeta2 : Inport  Port=5
  varpi : Inport  Port=6
  vartheta : Inport  Port=7
  Abs{2..7} (6 alike) : Abs  SaturateOnIntegerOverflow=off
  Demux{,1..6} (7 alike) : Demux  Outputs=3
  Divide1 : Product  Inputs=*/
  Divide2 : Product  Inputs=*/
  Divide3 : Product  Inputs=*/
  Mux : Mux  Inputs=3
  Power{2..7} (6 alike) : Math  Operator=pow
  Product{4..15} (12 alike) : Product
  Sign{2..7} (6 alike) : Signum
  Sum1 : Sum  Inputs=+++
  Sum2 : Sum  Inputs=+++
  Sum3 : Sum  Inputs=+++
  sigma_lineales : Outport
  wires:
  lambda/1 -> Demux2/1
  error_derivative/1 -> Demux1/1
  [vartheta_x] -> Divide1/2
  [varpi_x] -> Divide1/1
  Sum1/1 -> Mux/1
  varpi/1 -> Demux5/1
  Sum3/1 -> Mux/3
  Demux2/3 -> [lambda_z]
  Demux5/1 -> [varpi_x]
  Power2/1 -> Product4/1
  Demux/2 -> [error_y]
  Mux/1 -> sigma_lineales/1
  Demux4/3 -> [zeta2_z]
  Demux4/2 -> [zeta2_y]
  Demux4/1 -> [zeta2_x]
  Demux3/1 -> [zeta1_x]
  Demux3/2 -> [zeta1_y]
  Demux3/3 -> [zeta1_z]
  Demux6/2 -> [vartheta_y]
  Demux6/3 -> [vartheta_z]
  Demux6/1 -> [vartheta_x]
  [vartheta_z] -> Divide3/2
  [error_derivative_z] -> Abs7/1
  [error_derivative_z] -> Sign7/1
  Product11/1 -> Sum3/3
  [error_derivative_x] -> Abs3/1
  Power7/1 -> Product10/2
  Product10/1 -> Product11/1
  Divide3/1 -> Power7/2
  [error_z] -> Sum3/1
  [lambda_z] -> Power6/2
  [error_z] -> Sign6/1
  Sign7/1 -> Product11/2
  [zeta2_z] -> Product10/1
  Abs7/1 -> Power7/1
  Abs6/1 -> Power6/1
  Sign4/1 -> Product8/2
  Divide2/1 -> Power5/2
  vartheta/1 -> Demux6/1
  [lambda_y] -> Power4/2
  [error_derivative_y] -> Abs5/1
  Sign5/1 -> Product13/2
  Abs5/1 -> Power5/1
  [error_y] -> Sum2/1
  [zeta2_y] -> Product12/1
  [varpi_y] -> Divide2/1
  [zeta1_y] -> Product9/1
  Product14/1 -> Product15/2
  [zeta2_x] -> Product6/1
  Product8/1 -> Product9/2
  Product9/1 -> Sum2/2
  Product4/1 -> Product5/2
  Product7/1 -> Sum1/3
  [vartheta_y] -> Divide2/2
  Power4/1 -> Product8/1
  Sign3/1 -> Product7/2
  Power5/1 -> Product12/2
  Power6/1 -> Product14/1
  Abs2/1 -> Power2/1
  Power3/1 -> Product6/2
  Abs4/1 -> Power4/1
  Abs3/1 -> Power3/1
  [varpi_z] -> Divide3/1
  Sum2/1 -> Mux/2
  [error_x] -> Sum1/1
  [error_y] -> Sign4/1
  [zeta1_x] -> Product5/1
  Sign6/1 -> Product14/2
  Demux5/2 -> [varpi_y]
  Product5/1 -> Sum1/2
  Demux5/3 -> [varpi_z]
  Product12/1 -> Product13/1
  Product15/1 -> Sum3/2
  zeta2/1 -> Demux4/1
  Demux1/1 -> [error_derivative_x]
  Divide1/1 -> Power3/2
  Sign2/1 -> Product4/2
  [zeta1_z] -> Product15/1
  Demux1/3 -> [error_derivative_z]
  [error_z] -> Abs6/1
  [error_x] -> Sign2/1
  Demux/1 -> [error_x]
  Demux/3 -> [error_z]
  [error_y] -> Abs4/1
  [error_derivative_x] -> Sign3/1
  Product6/1 -> Product7/1
  Demux1/2 -> [error_derivative_y]
  error1/1 -> Demux/1
  Product13/1 -> Sum2/3
  Demux2/2 -> [lambda_y]
  [error_derivative_y] -> Sign5/1
  Demux2/1 -> [lambda_x]
  zeta1/1 -> Demux3/1
  [error_x] -> Abs2/1
  [lambda_x] -> Power2/2

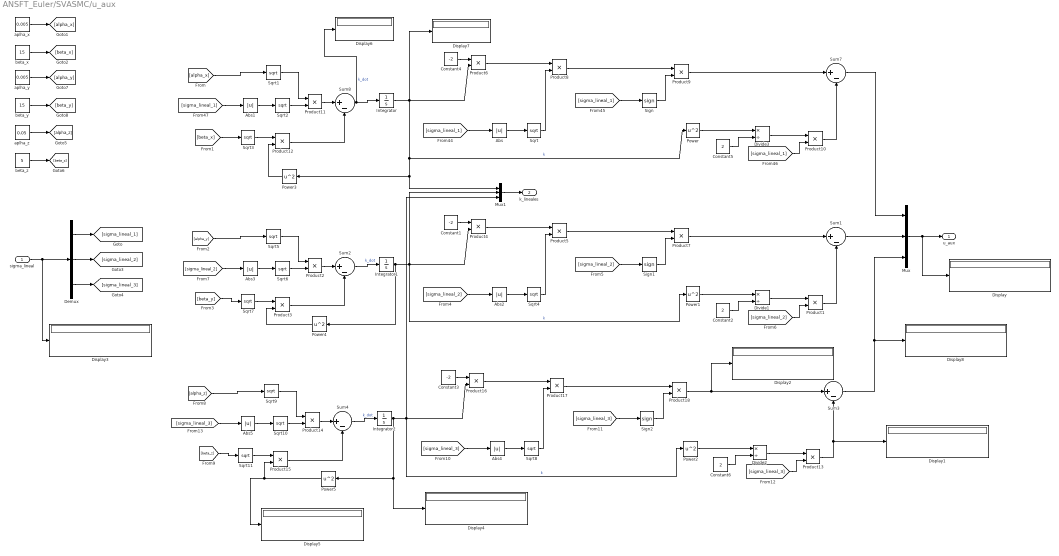
== system ANSFT_Euler/SVASMC/u_aux ==
  sigma_lineal : Inport
  Abs{,1..5} (6 alike) : Abs  SaturateOnIntegerOverflow=off
  Constant1 : Constant  Value=-2
  Constant2 : Constant  Value=2
  Constant3 : Constant  Value=-2
  Constant4 : Constant  Value=-2
  Constant5 : Constant  Value=2
  Constant6 : Constant  Value=2
  Demux : Demux  Outputs=3
  Display{,1..8} (9 alike) : Display
  Divide1 : Product  Inputs=*/
  Divide2 : Product  Inputs=*/
  Divide3 : Product  Inputs=*/
  Integrator : Integrator
  Integrator1 : Integrator
  Integrator2 : Integrator
  Mux : Mux  Inputs=3
  Mux1 : Mux  Inputs=3
  Power{,1..5} (6 alike) : Math  Operator=square
  Product{1..18} (18 alike) : Product
  Sign : Signum
  Sign1 : Signum
  Sign2 : Signum
  Sqrt{,1..11} (12 alike) : Sqrt
  Sum{1..4,7..8} (6 alike) : Sum  Inputs=|+-
  aplha_x : Constant  Value=0.005
  aplha_y : Constant  Value=0.005
  aplha_z : Constant  Value=0.05
  beta_x : Constant  Value=15
  beta_y : Constant  Value=15
  beta_z : Constant  Value=5
  u_aux : Outport
  k_lineales : Outport  Port=2
  wires:
  Constant5/1 -> Divide3/2
  Sqrt3/1 -> Product12/1
  [sigma_lineal_1] -> Abs1/1
  Sign/1 -> Product9/2
  Product10/1 -> Sum7/2
  Constant4/1 -> Product6/1
  Product8/1 -> Product9/1
  Abs/1 -> Sqrt/1
  [sigma_lineal_1] -> Abs/1
  Divide3/1 -> Product10/1
  Product6/1 -> Product8/1
  [sigma_lineal_1] -> Product10/2
  Abs1/1 -> Sqrt2/1
  Sqrt1/1 -> Product11/1
  [sigma_lineal_1] -> Sign/1
  Product9/1 -> Sum7/1
  Product12/1 -> Sum8/2
  Product11/1 -> Sum8/1
  Sqrt/1 -> Product8/2
  Integrator/1 -> Mux1/1, Power3/1, Power/1, Display7/1, Product6/2  "k"
  Power/1 -> Divide3/1
  Sum8/1 -> Display6/1, Integrator/1  "k_dot"
  Sqrt2/1 -> Product11/2
  sigma_lineal/1 -> Display3/1, Demux/1
  Demux/1 -> [sigma_lineal_1]
  aplha_x/1 -> [alpha_x]
  [alpha_x] -> Sqrt1/1
  beta_x/1 -> [beta_x]
  [beta_x] -> Sqrt3/1
  Demux/2 -> [sigma_lineal_2]
  Demux/3 -> [sigma_lineal_3]
  [beta_y] -> Sqrt7/1
  [alpha_y] -> Sqrt5/1
  Sqrt6/1 -> Product2/2
  Sum2/1 -> Integrator1/1  "k_dot"
  Power1/1 -> Divide1/1
  Integrator1/1 -> Mux1/2, Power1/1, Product4/2, Power4/1  "k"
  Sqrt4/1 -> Product5/2
  Product2/1 -> Sum2/1
  Product3/1 -> Sum2/2
  Product7/1 -> Sum1/1
  [sigma_lineal_2] -> Sign1/1
  Sqrt5/1 -> Product2/1
  Abs3/1 -> Sqrt6/1
  [sigma_lineal_2] -> Product1/2
  Product4/1 -> Product5/1
  Divide1/1 -> Product1/1
  [sigma_lineal_2] -> Abs2/1
  Abs2/1 -> Sqrt4/1
  Product5/1 -> Product7/1
  Constant1/1 -> Product4/1
  Product1/1 -> Sum1/2
  Sign1/1 -> Product7/2
  [sigma_lineal_2] -> Abs3/1
  Sqrt7/1 -> Product3/1
  Constant2/1 -> Divide1/2
  Sum3/1 -> Display8/1, Mux/3
  Constant6/1 -> Divide2/2
  Sqrt11/1 -> Product15/1
  [sigma_lineal_3] -> Abs5/1
  Sign2/1 -> Product18/2
  Product13/1 -> Display1/1, Sum3/2
  Constant3/1 -> Product16/1
  Product17/1 -> Product18/1
  Abs4/1 -> Sqrt8/1
  [sigma_lineal_3] -> Abs4/1
  Divide2/1 -> Product13/1
  Product16/1 -> Product17/1
  [sigma_lineal_3] -> Product13/2
  Abs5/1 -> Sqrt10/1
  Sqrt9/1 -> Product14/1
  [sigma_lineal_3] -> Sign2/1
  Product18/1 -> Display2/1, Sum3/1
  Product15/1 -> Sum4/2
  Product14/1 -> Sum4/1
  Sqrt8/1 -> Product17/2
  Integrator2/1 -> Display4/1, Power5/1, Mux1/3, Product16/2, Power2/1  "k"
  Power2/1 -> Divide2/1
  Sum4/1 -> Integrator2/1  "k_dot"
  Sqrt10/1 -> Product14/2
  [alpha_z] -> Sqrt9/1
  [beta_z] -> Sqrt11/1
  Mux/1 -> Display/1, u_aux/1
  Power3/1 -> Product12/2
  Power4/1 -> Product3/2
  Power5/1 -> Display5/1, Product15/2
  beta_z/1 -> [beta_z]
  aplha_z/1 -> [alpha_z]
  beta_y/1 -> [beta_y]
  aplha_y/1 -> [alpha_y]
  Mux1/1 -> k_lineales/1
  Sum7/1 -> Mux/1
  Sum1/1 -> Mux/2

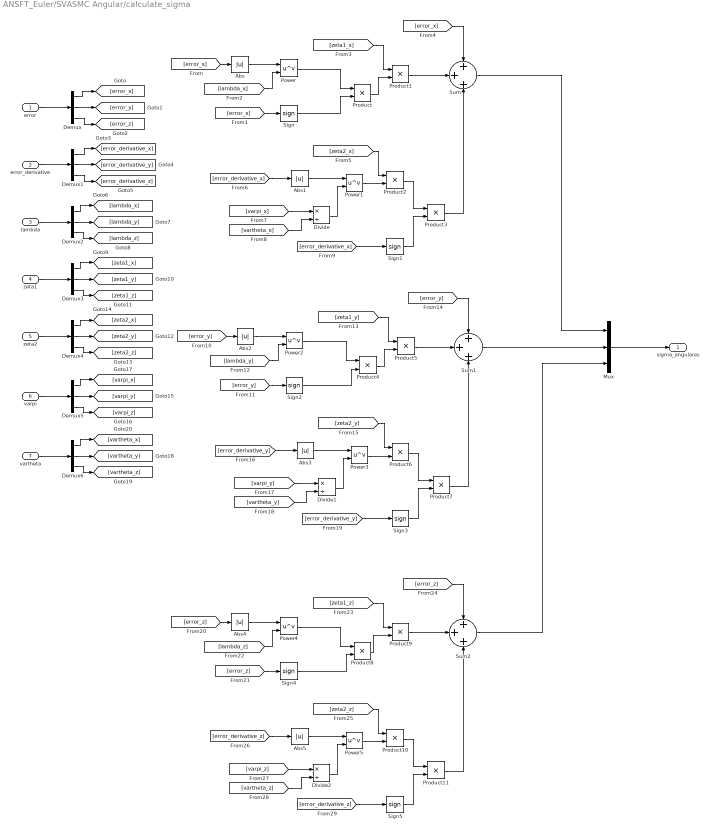
== system ANSFT_Euler/SVASMC Angular/calculate_sigma ==
  error : Inport
  error_derivative : Inport  Port=2
  lambda : Inport  Port=3
  zeta1 : Inport  Port=4
  zeta2 : Inport  Port=5
  varpi : Inport  Port=6
  vartheta : Inport  Port=7
  Abs{,1..5} (6 alike) : Abs  SaturateOnIntegerOverflow=off
  Demux{,1..6} (7 alike) : Demux  Outputs=3
  Divide : Product  Inputs=*/
  Divide1 : Product  Inputs=*/
  Divide2 : Product  Inputs=*/
  Mux : Mux  Inputs=3
  Power{,1..5} (6 alike) : Math  Operator=pow
  Product{,1..11} (12 alike) : Product
  Sign{,1..5} (6 alike) : Signum
  Sum : Sum  Inputs=+++
  Sum1 : Sum  Inputs=+++
  Sum2 : Sum  Inputs=+++
  sigma_angulares : Outport
  wires:
  Abs/1 -> Power/1
  Sign/1 -> Product/2
  Product/1 -> Product1/2
  Product1/1 -> Sum/2
  Abs1/1 -> Power1/1
  Divide/1 -> Power1/2
  Power1/1 -> Product2/2
  Sign1/1 -> Product3/2
  Product2/1 -> Product3/1
  Product3/1 -> Sum/3
  Power/1 -> Product/1
  error/1 -> Demux/1
  error_derivative/1 -> Demux1/1
  lambda/1 -> Demux2/1
  Demux/1 -> [error_x]
  Demux/2 -> [error_y]
  Demux/3 -> [error_z]
  Demux1/1 -> [error_derivative_x]
  Demux1/2 -> [error_derivative_y]
  Demux1/3 -> [error_derivative_z]
  Demux2/1 -> [lambda_x]
  Demux2/2 -> [lambda_y]
  Demux2/3 -> [lambda_z]
  Demux3/3 -> [zeta1_z]
  Demux3/2 -> [zeta1_y]
  Demux3/1 -> [zeta1_x]
  zeta1/1 -> Demux3/1
  zeta2/1 -> Demux4/1
  Demux4/1 -> [zeta2_x]
  Demux4/2 -> [zeta2_y]
  Demux4/3 -> [zeta2_z]
  Demux5/3 -> [varpi_z]
  Demux5/2 -> [varpi_y]
  Demux5/1 -> [varpi_x]
  varpi/1 -> Demux5/1
  vartheta/1 -> Demux6/1
  Demux6/1 -> [vartheta_x]
  Demux6/2 -> [vartheta_y]
  Demux6/3 -> [vartheta_z]
  [error_x] -> Abs/1
  [error_x] -> Sign/1
  [lambda_x] -> Power/2
  [zeta1_x] -> Product1/1
  [error_x] -> Sum/1
  [zeta2_x] -> Product2/1
  [error_derivative_x] -> Abs1/1
  [varpi_x] -> Divide/1
  [vartheta_x] -> Divide/2
  [error_derivative_x] -> Sign1/1
  Sum/1 -> Mux/1
  Mux/1 -> sigma_angulares/1
  [error_derivative_y] -> Sign3/1
  [vartheta_y] -> Divide1/2
  [varpi_y] -> Divide1/1
  [error_derivative_y] -> Abs3/1
  [zeta2_y] -> Product6/1
  [error_y] -> Sum1/1
  [zeta1_y] -> Product5/1
  [lambda_y] -> Power2/2
  [error_y] -> Sign2/1
  [error_y] -> Abs2/1
  Power2/1 -> Product4/1
  Product7/1 -> Sum1/3
  Product6/1 -> Product7/1
  Sign3/1 -> Product7/2
  Power3/1 -> Product6/2
  Divide1/1 -> Power3/2
  Abs3/1 -> Power3/1
  Product5/1 -> Sum1/2
  Product4/1 -> Product5/2
  Sign2/1 -> Product4/2
  Abs2/1 -> Power2/1
  Sum1/1 -> Mux/2
  Sum2/1 -> Mux/3
  Abs4/1 -> Power4/1
  Sign4/1 -> Product8/2
  Product8/1 -> Product9/2
  Product9/1 -> Sum2/2
  Abs5/1 -> Power5/1
  Divide2/1 -> Power5/2
  Power5/1 -> Product10/2
  Sign5/1 -> Product11/2
  Product10/1 -> Product11/1
  Product11/1 -> Sum2/3
  Power4/1 -> Product8/1
  [error_z] -> Abs4/1
  [error_z] -> Sign4/1
  [lambda_z] -> Power4/2
  [zeta1_z] -> Product9/1
  [error_z] -> Sum2/1
  [zeta2_z] -> Product10/1
  [error_derivative_z] -> Abs5/1
  [varpi_z] -> Divide2/1
  [vartheta_z] -> Divide2/2
  [error_derivative_z] -> Sign5/1

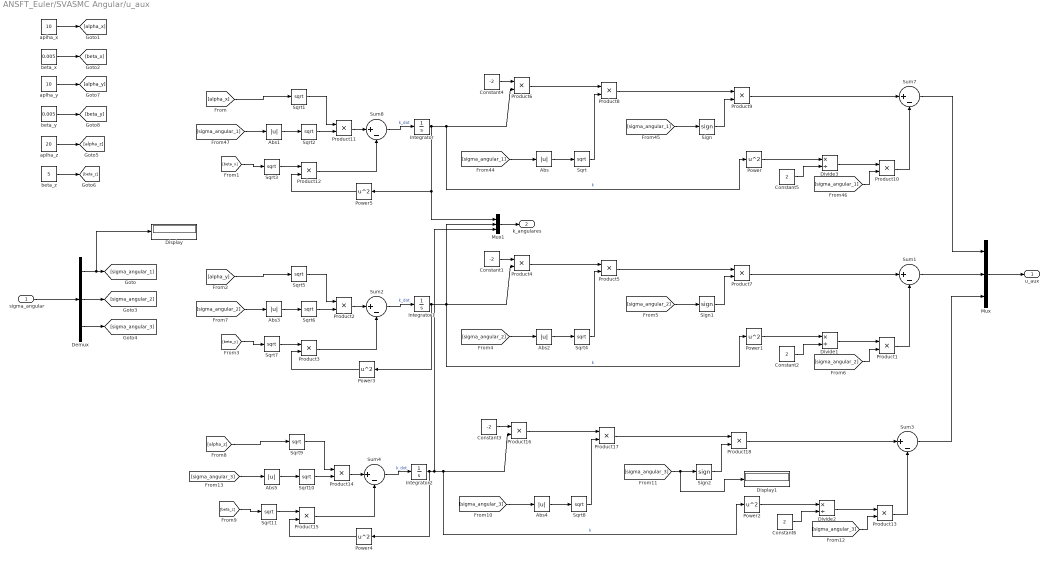
== system ANSFT_Euler/SVASMC Angular/u_aux ==
  sigma_angular : Inport
  Abs{,1..5} (6 alike) : Abs  SaturateOnIntegerOverflow=off
  Constant1 : Constant  Value=-2
  Constant2 : Constant  Value=2
  Constant3 : Constant  Value=-2
  Constant4 : Constant  Value=-2
  Constant5 : Constant  Value=2
  Constant6 : Constant  Value=2
  Demux : Demux  Outputs=3
  Display : Display
  Display1 : Display
  Divide1 : Product  Inputs=*/
  Divide2 : Product  Inputs=*/
  Divide3 : Product  Inputs=*/
  Integrator : Integrator
  Integrator1 : Integrator
  Integrator2 : Integrator
  Mux : Mux  Inputs=3
  Mux1 : Mux  Inputs=3
  Power{,1..5} (6 alike) : Math  Operator=square
  Product{1..18} (18 alike) : Product
  Sign : Signum
  Sign1 : Signum
  Sign2 : Signum
  Sqrt{,1..11} (12 alike) : Sqrt
  Sum{1..4,7..8} (6 alike) : Sum  Inputs=|+-
  aplha_x : Constant  Value=10
  aplha_y : Constant  Value=10
  aplha_z : Constant  Value=20
  beta_x : Constant  Value=0.005
  beta_y : Constant  Value=0.005
  beta_z : Constant  Value=5
  u_aux : Outport
  k_angulares : Outport  Port=2
  wires:
  Constant5/1 -> Divide3/2
  Sqrt3/1 -> Product12/1
  [sigma_angular_1] -> Abs1/1
  Sign/1 -> Product9/2
  Product10/1 -> Sum7/2
  Constant4/1 -> Product6/1
  Product8/1 -> Product9/1
  Abs/1 -> Sqrt/1
  [sigma_angular_1] -> Abs/1
  Divide3/1 -> Product10/1
  Product6/1 -> Product8/1
  [sigma_angular_1] -> Product10/2
  Abs1/1 -> Sqrt2/1
  Sqrt1/1 -> Product11/1
  [sigma_angular_1] -> Sign/1
  Product9/1 -> Sum7/1
  Product12/1 -> Sum8/2
  Product11/1 -> Sum8/1
  Sqrt/1 -> Product8/2
  Integrator/1 -> Mux1/1, Power5/1, Product6/2, Power/1  "k"
  Power/1 -> Divide3/1
  Sum8/1 -> Integrator/1  "k_dot"
  Sqrt2/1 -> Product11/2
  sigma_angular/1 -> Demux/1
  Demux/1 -> Display/1, [sigma_angular_1]
  [alpha_x] -> Sqrt1/1
  [beta_x] -> Sqrt3/1
  Demux/2 -> [sigma_angular_2]
  Demux/3 -> [sigma_angular_3]
  [beta_y] -> Sqrt7/1
  [alpha_y] -> Sqrt5/1
  Sqrt6/1 -> Product2/2
  Sum2/1 -> Integrator1/1  "k_dot"
  Power1/1 -> Divide1/1
  Integrator1/1 -> Mux1/2, Power1/1, Product4/2, Power3/1  "k"
  Sqrt4/1 -> Product5/2
  Product2/1 -> Sum2/1
  Product3/1 -> Sum2/2
  Product7/1 -> Sum1/1
  [sigma_angular_2] -> Sign1/1
  Sqrt5/1 -> Product2/1
  Abs3/1 -> Sqrt6/1
  [sigma_angular_2] -> Product1/2
  Product4/1 -> Product5/1
  Divide1/1 -> Product1/1
  [sigma_angular_2] -> Abs2/1
  Abs2/1 -> Sqrt4/1
  Product5/1 -> Product7/1
  Constant1/1 -> Product4/1
  Product1/1 -> Sum1/2
  Sign1/1 -> Product7/2
  [sigma_angular_2] -> Abs3/1
  Sqrt7/1 -> Product3/1
  Constant2/1 -> Divide1/2
  Sum1/1 -> Mux/2
  Sum3/1 -> Mux/3
  Constant6/1 -> Divide2/2
  Sqrt11/1 -> Product15/1
  [sigma_angular_3] -> Abs5/1
  Sign2/1 -> Product18/2
  Product13/1 -> Sum3/2
  Constant3/1 -> Product16/1
  Product17/1 -> Product18/1
  Abs4/1 -> Sqrt8/1
  [sigma_angular_3] -> Abs4/1
  Divide2/1 -> Product13/1
  Product16/1 -> Product17/1
  [sigma_angular_3] -> Product13/2
  Abs5/1 -> Sqrt10/1
  Sqrt9/1 -> Product14/1
  [sigma_angular_3] -> Display1/1, Sign2/1
  Product18/1 -> Sum3/1
  Product15/1 -> Sum4/2
  Product14/1 -> Sum4/1
  Sqrt8/1 -> Product17/2
  Integrator2/1 -> Power4/1, Mux1/3, Product16/2, Power2/1  "k"
  Power2/1 -> Divide2/1
  Sum4/1 -> Integrator2/1  "k_dot"
  Sqrt10/1 -> Product14/2
  [alpha_z] -> Sqrt9/1
  [beta_z] -> Sqrt11/1
  Sum7/1 -> Mux/1
  Mux/1 -> u_aux/1
  Power5/1 -> Product12/2
  Power3/1 -> Product3/2
  Power4/1 -> Product15/2
  beta_x/1 -> [beta_x]
  aplha_x/1 -> [alpha_x]
  beta_z/1 -> [beta_z]
  aplha_y/1 -> [alpha_y]
  aplha_z/1 -> [alpha_z]
  beta_y/1 -> [beta_y]
  Mux1/1 -> k_angulares/1

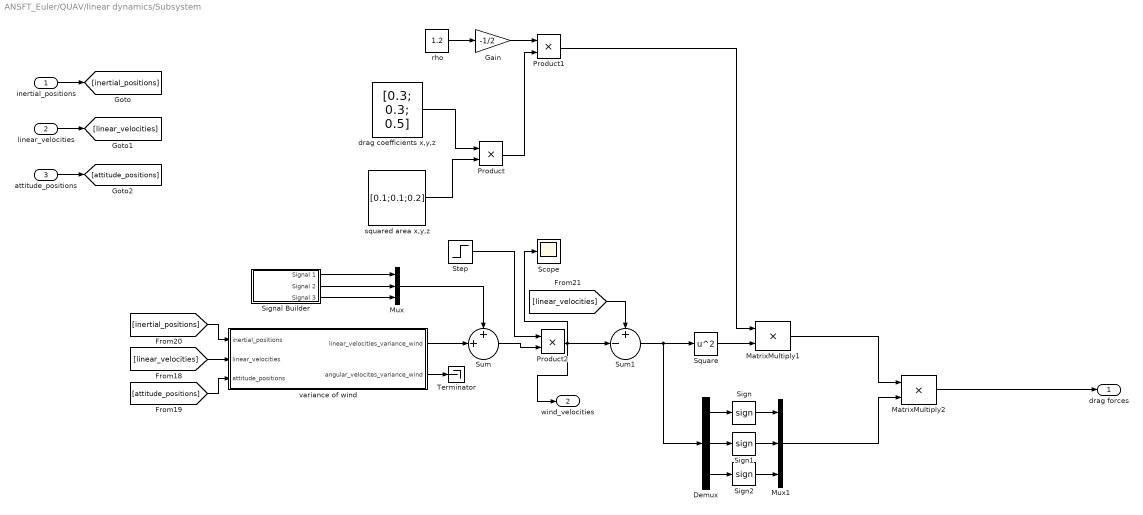
== system ANSFT_Euler/QUAV/linear dynamics/Subsystem ==
  inertial_positions : Inport
  linear_velocities : Inport  Port=2
  attitude_positions : Inport  Port=3
  Demux : Demux  Outputs=3
  Gain : Gain  Gain=-1/2
  MatrixMultiply1 : Product
  MatrixMultiply2 : Product
  Mux : Mux  Inputs=3
  Mux1 : Mux  Inputs=3
  Product : Product
  Product1 : Product
  Product2 : Product
  Scope : Scope
  Sign : Signum
  Sign1 : Signum
  Sign2 : Signum
  Signal Builder : Subsystem  Tag=STV Subsys  LoadFcn=sigbuilder_block('load');  StartFcn=sigbuilder_block('start');  StopFcn=sigbuilder_block('stop');  ClipboardFcn=sigbuilder_block('clipboard');  mask(Sigbuilder block){tuvar=[0:10]}
      mask help: Simulink:masks:SigbuilderBlock_MD
      mask init:
      | if ~strcmp(get_param(bdroot(gcbh),'SimulationStatus'),'stopped') tuvar = sigbuilder_block('maskInit'); end
      settings: CopyFcn=sigbuilder_block('copy');  DeleteFcn=sigbuilder_block('delete');  ModelCloseFcn=sigbuilder_block('modelClose');  PreSaveFcn=sigbuilder_block('preSave');  PauseFcn=sigbuilder_block('pause');  ContinueFcn=sigbuilder_block('continue');  NameChangeFcn=sigbuilder_block('namechange');  OpenFcn=sigbuilder_block('open',[53.4433 0 1371.71 713.32 ]);  CloseFcn=sigbuilder_block('close');
      mask Display: plot(0, 0, 100, 100,[2, 2, 32, 32, 2], [68, 8, 8, 68, 68],[32, 2], [38, 38], [32, 19, 2],[53, 60, 44], [32, 17, 17, 2],[16, 16, 31, 31]);txt = getActiveGroup(gcbh);text(2, 100, txt,'verticalAlignment', 'top');
  Square : Math  Operator=square
  Step : Step  Time=15  SampleTime=0
  Sum : Sum  Inputs=++|
  Sum1 : Sum  Inputs=+-|
  Terminator : Terminator
  drag coefficients x,y,z : Constant  Value=[0.3; 0.3; 0.5]  VectorParams1D=off
  rho : Constant  Value=1.2
  squared area x,y,z : Constant  Value=[0.1;0.1;0.2]  VectorParams1D=off
  variance of wind : Subsystem
  "drag forces " : Outport
  wind_velocities : Outport  Port=2
  wires:
  Demux/1 -> Sign/1
  Product1/1 -> MatrixMultiply1/1
  [attitude_positions] -> variance of wind/3(attitude_positions)
  Sign/1 -> Mux1/1
  Demux/3 -> Sign2/1
  Square/1 -> MatrixMultiply1/2
  Demux/2 -> Sign1/1
  MatrixMultiply1/1 -> MatrixMultiply2/1
  Sign1/1 -> Mux1/2
  variance of wind/2(angular_velocites_variance_wind) -> Terminator/1
  [inertial_positions] -> variance of wind/1(inertial_positions)
  Gain/1 -> Product1/1
  rho/1 -> Gain/1
  [linear_velocities] -> variance of wind/2(linear_velocities)
  variance of wind/1(linear_velocities_variance_wind) -> Sum/2
  Mux/1 -> Sum/1
  Mux1/1 -> MatrixMultiply2/2
  [linear_velocities] -> Sum1/1
  Product/1 -> Product1/2
  Sign2/1 -> Mux1/3
  Sum1/1 -> Square/1, Demux/1
  drag coefficients x,y,z/1 -> Product/1
  inertial_positions/1 -> [inertial_positions]
  linear_velocities/1 -> [linear_velocities]
  attitude_positions/1 -> [attitude_positions]
  MatrixMultiply2/1 -> "drag forces "/1
  squared area x,y,z/1 -> Product/2
  Signal Builder/1(Signal 1) -> Mux/1
  Signal Builder/2(Signal 2) -> Mux/2
  Signal Builder/3(Signal 3) -> Mux/3
  Sum/1 -> Product2/2
  Product2/1 -> wind_velocities/1, Sum1/2, Scope/1
  Step/1 -> Product2/1

== system ANSFT_Euler/QUAV/linear dynamics/Subsystem/Signal Builder ==
  Demux : Demux  Tag=STV Demux  Outputs=3
      settings: DisplayOption=none
  FromWs : FromWorkspace  Tag=STV FromWs  VariableName=tuvar
      SigBuilderData=|
      | common.afterFinalStr = 'Extrapolate'
      | common.sampleTime = 0
      | dataSet.timeRange = [0 200]
      | dataSet.name = 'Group 1'
      | sbobj.Groups.Name = 'Group 1'
      | sbobj.Groups.Signals(1).Name = 'Signal 1'
      | sbobj.Groups.Signals(1).XData = [0 1 2 3 4 5 6 7 8 9 10 11 12 13 14 15 16 17 18 19 20 21 22 23 24 25 26 27 28 29 30 31 32 33 34 35 36 37 38 39 40 41 42 43 44 45 46 47 48 49 50 51 52 53 54 55 56 57 58 59 60 61 62 63 64 65 66 67 68 69 70 71 72 73 74 75 76 77 78 79 80 81 82 83 84 85 86 87 88 89 90 91 92 93 94 95 96 97 98 99 100 101 102 103 104 105 106 107 108 109 110 111 112 113 114 115 116 117 118 119 120 121 122 123 124 125 126 127 128 129 130 131 132 133 134 135 136 137 138 139 140 141 142 143 144 145 146 147 148 149 150 151 152 153 154 155 156 157 158 159 160 161 162 163 164 165 166 167 168 169 170 171 172 173 174 175 176 177 178 179 180 181 182 183 184 185 186 187 188 189 190 191 192 193 194 195 196 197 198 199 200]
      | sbobj.Groups.Signals(1).YData = [4.99289151409 6.23556959864 9.65695909959 6.77285589819 4.5118290285 1.05375596505 5.49812022791 5.52195500679 3.41703862854 7.0186665157 5.7817454464 6.17380071378 ... (201 elements, 1x201)]
      | sbobj.Groups.Signals(2).Name = 'Signal 2'
      | sbobj.Groups.Signals(2).XData = [0 1 2 3 4 5 6 7 8 9 10 11 12 13 14 15 16 17 18 19 20 21 22 23 24 25 26 27 28 29 30 31 32 33 34 35 36 37 38 39 40 41 42 43 44 45 46 47 48 49 50 51 52 53 54 55 56 57 58 59 60 61 62 63 64 65 66 67 68 69 70 71 72 73 74 75 76 77 78 79 80 81 82 83 84 85 86 87 88 89 90 91 92 93 94 95 96 97 98 99 100 101 102 103 104 105 106 107 108 109 110 111 112 113 114 115 116 117 118 119 120 121 122 123 124 125 126 127 128 129 130 131 132 133 134 135 136 137 138 139 140 141 142 143 144 145 146 147 148 149 150 151 152 153 154 155 156 157 158 159 160 161 162 163 164 165 166 167 168 169 170 171 172 173 174 175 176 177 178 179 180 181 182 183 184 185 186 187 188 189 190 191 192 193 194 195 196 197 198 199 200]
      | sbobj.Groups.Signals(2).YData = [5.48956735199 2.95949128858 7.25568136366 9.46493740303 3.45150581312 2.99708542708 7.2766526975 4.95209682258 2.27233540889 7.47263236681 4.69184931229 3.40958682702 ... (201 elements, 1x201)]
      | sbobj.Groups.Signals(3).Name = 'Signal 3'
      | sbobj.Groups.Signals(3).XData = [0 1 2 3 4 5 6 7 8 9 10 11 12 13 14 15 16 17 18 19 20 21 22 23 24 25 26 27 28 29 30 31 32 33 34 35 36 37 38 39 40 41 42 43 44 45 46 47 48 49 50 51 52 53 54 55 56 57 58 59 60 61 62 63 64 65 66 67 68 69 70 71 72 73 74 75 76 77 78 79 80 81 82 83 84 85 86 87 88 89 90 91 92 93 94 95 96 97 98 99 100 101 102 103 104 105 106 107 108 109 110 111 112 113 114 115 116 117 118 119 120 121 122 123 124 125 126 127 128 129 130 131 132 133 134 135 136 137 138 139 140 141 142 143 144 145 146 147 148 149 150 151 152 153 154 155 156 157 158 159 160 161 162 163 164 165 166 167 168 169 170 171 172 173 174 175 176 177 178 179 180 181 182 183 184 185 186 187 188 189 190 191 192 193 194 195 196 197 198 199 200]
      | sbobj.Groups.Signals(3).YData = [0.584923384066 1.75613099095 2.04025070079 0.626170570198 3.07918731484 2.7439311595 3.5428606501 2.68752214674 -1.5501683039 1.0329468474 2.3117904282 1.18493105713 ... (201 elements, 1x201)]
      | sbobj.Groups.TimeRange = [0 200]
  Signal 1 : Outport  Tag=STV Outport
  Signal 2 : Outport  Tag=STV Outport  Port=2
  Signal 3 : Outport  Tag=STV Outport  Port=3
  wires:
  FromWs/1 -> Demux/1
  Demux/1 -> Signal 1/1
  Demux/2 -> Signal 2/1
  Demux/3 -> Signal 3/1
